simulink model "Test"  (R2026a)
settings: Solver=FixedStepDiscrete  FixedStep=1/200
undefined symbols (not defined in the file or in its folder): position, timestamp, x, y, z
libraries: px4_lib x33, dspsigops x3
settings Model: Creator=jack  LastModifiedBy=jack
settings OptimizationCC: DefaultUnderspecifiedDataType=single
settings DebuggingCC: ParameterPrecisionLossMsg=none
settings HardwareCC: ProdBitPerLong=64.0  ProdHWDeviceType=Intel->x86-64 (Linux 64)
settings SFSimCC: SimCustomHeaderCode="#include \"px4_simulink_api.h\""  SimUserSources=px4_simulink_api.cpp  SimTargetLang=C++
settings RTWCC: SystemTargetFile=ert.tlc  GenCodeOnly=on  PostCodeGenCommand=px4API.runPostCodeGen(buildInfo)  CustomHeaderCode="#include \"px4_simulink_api.h\""  Toolchain=GNU Tools for PX4 Autopilots  DataTypeReplacement=CDataTypesFixedWidth  TargetLang=C++  Description=Embedded Coder
settings ERTTargetCC: ExtModeTransport=2.0  RootIOFormat=Structure reference  MaxIdInt64=INT64_MAX  MinIdInt64=INT64_MIN  MaxIdUint64=UINT64_MAX  MaxIdInt32=INT32_MAX  MinIdInt32=INT32_MIN  MaxIdUint32=UINT32_MAX  MaxIdInt16=INT16_MAX  MinIdInt16=INT16_MIN  MaxIdUint16=UINT16_MAX  MaxIdInt8=INT8_MAX  MinIdInt8=INT8_MIN  MaxIdUint8=UINT8_MAX  TargetLangStandard=C++14 (ISO)  CodeInterfacePackaging=C++ class  SubcomponentCodeInterfacePackaging=C++ class

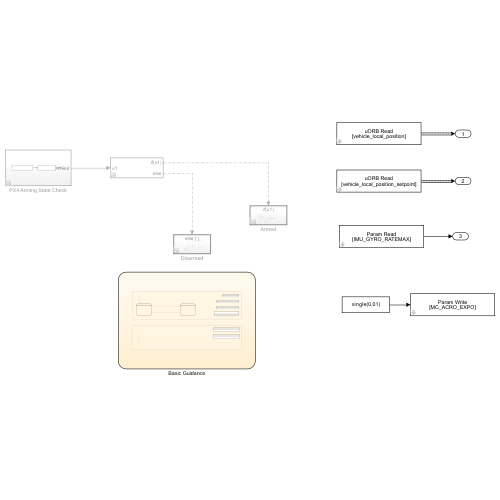
[thumbnail: Simulink's stored preview of the top-level diagram]
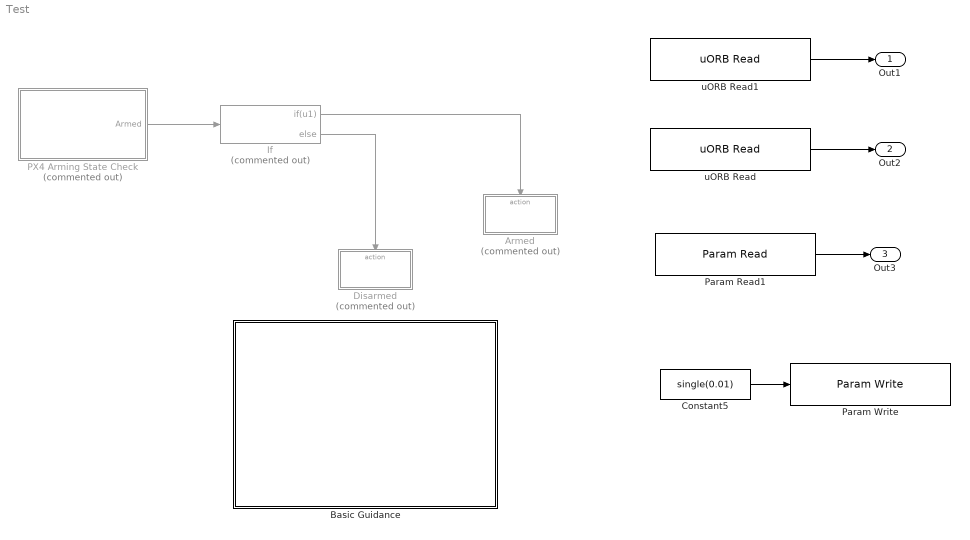
== system Test ==
  Armed : Subsystem  Commented=on  TreatAsAtomicUnit=on
  Basic Guidance : Stateflow chart  TreatAsAtomicUnit=on
  Constant5 : Constant  Value=single(0.01)
  Disarmed : Subsystem  Commented=on  TreatAsAtomicUnit=on
  If : If  Commented=on  IfExpression=u1
  PX4 Arming State Check : Subsystem  Commented=on
  Param Read1 : px4_lib/Param Read  param_name=IMU_GYRO_RATEMAX  param_type=int32  sample_time=-1
  Param Write : px4_lib/Param Write  param_name=MC_ACRO_EXPO  param_type=single  sample_time=1/5
  uORB Read : px4_lib/uORB Read  uorb_topic=vehicle_local_position_setpoint  sample_time=1/200
  uORB Read1 : px4_lib/uORB Read  uorb_topic=vehicle_local_position  sample_time=1/200
  Out1 : Outport
  Out2 : Outport  Port=2
  Out3 : Outport  Port=3
  wires:
  uORB Read1/1 -> Out1/1
  uORB Read/1 -> Out2/1
  Param Read1/1 -> Out3/1
  Constant5/1 -> Param Write/1
  PX4 Arming State Check/1(Armed) -> If/1
  If/1 -> Armed/Action
  If/2 -> Disarmed/Action

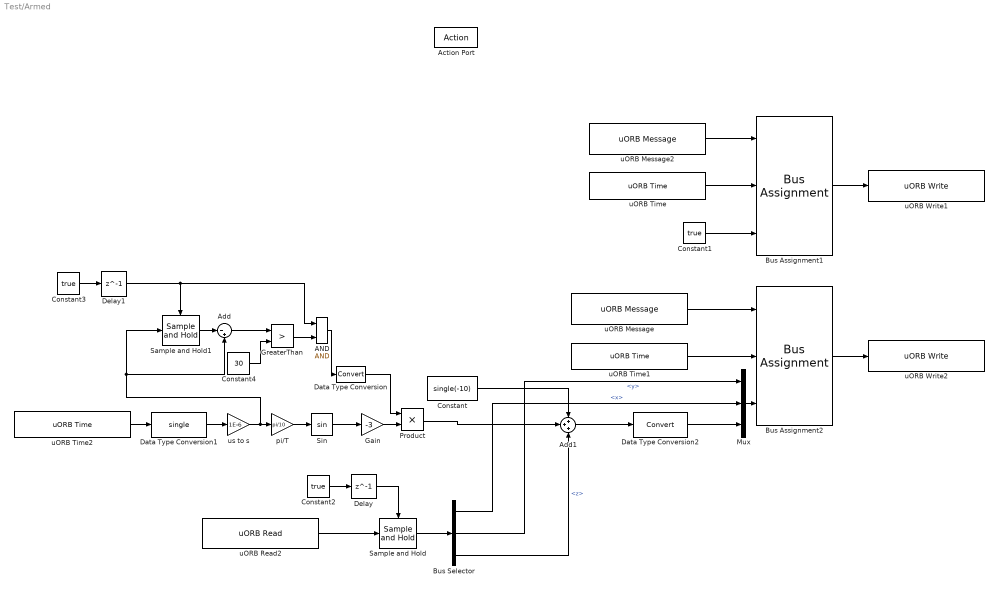
== system Test/Armed ==
  Action Port : ActionPort  InitializeStates=reset  ActionPortLabel=if(u1)
  AND : Logic  IconShape=distinctive  AllPortsSameDT=off  OutDataTypeStr=boolean
  Add : Sum  Inputs=|-+
  Add1 : Sum  Inputs=+++
  Bus Assignment1 : BusAssignment  AssignedSignals=timestamp,position
  Bus Assignment2 : BusAssignment  AssignedSignals=timestamp,position
  Bus Selector : BusSelector  OutputSignals=x,y,z
  Constant : Constant  Value=single(-10)
  Constant1 : Constant  Value=true
  Constant2 : Constant  Value=true
  Constant3 : Constant  Value=true
  Constant4 : Constant  Value=30
  Data Type Conversion : DataTypeConversion  SaturateOnIntegerOverflow=off  RndMeth=Floor
  Data Type Conversion1 : DataTypeConversion  OutDataTypeStr=single  SaturateOnIntegerOverflow=off  RndMeth=Floor
  Data Type Conversion2 : DataTypeConversion  SaturateOnIntegerOverflow=off  RndMeth=Floor
  Delay : Delay  DelayLength=1  InitialCondition=false
  Delay1 : Delay  DelayLength=1  InitialCondition=false
  Gain : Gain  Gain=-3  ParamDataTypeStr=single
  GreaterThan : RelationalOperator  Operator=>  OutDataTypeStr=boolean  RndMeth=Simplest  InputSameDT=off
  Mux : Mux  Inputs=3
  Product : Product
  Sample and Hold : dspsigops/Sample and Hold  trig=Rising edge  initCond=0  latchinput=off
  Sample and Hold1 : dspsigops/Sample and Hold  trig=Rising edge  initCond=0  latchinput=off
  Sin : Trigonometry  OutputSignalType=real
  pi/T : Gain  Gain=pi/10  ParamDataTypeStr=single
  uORB Message : px4_lib/uORB Message  uorb_topic=trajectory_setpoint6dof  sample_time=-1  init_value=NaN
  uORB Message2 : px4_lib/uORB Message  uorb_topic=offboard_control_mode  sample_time=-1  init_value=0
  uORB Read2 : px4_lib/uORB Read  uorb_topic=vehicle_local_position_setpoint  sample_time=-1
  uORB Time : px4_lib/uORB Time  sample_time=-1
  uORB Time1 : px4_lib/uORB Time  sample_time=-1
  uORB Time2 : px4_lib/uORB Time  sample_time=-1
  uORB Write1 : px4_lib/uORB Write  uorb_topic=offboard_control_mode  sample_time=1/50
  uORB Write2 : px4_lib/uORB Write  uorb_topic=vehicle_local_position_setpoint  sample_time=1/50
  us to s : Gain  Gain=1E-6  ParamDataTypeStr=single
  wires:
  uORB Message/1 -> Bus Assignment2/1
  uORB Time/1 -> Bus Assignment1/2
  Bus Selector/3 -> Add1/3  "<z>"
  Bus Selector/2 -> Mux/1  "<y>"
  Mux/1 -> Bus Assignment2/3
  uORB Time1/1 -> Bus Assignment2/2
  pi/T/1 -> Sin/1
  Constant/1 -> Add1/1
  Gain/1 -> Product/2
  Bus Assignment1/1 -> uORB Write1/1
  uORB Message2/1 -> Bus Assignment1/1
  GreaterThan/1 -> AND/2
  Constant2/1 -> Delay/1
  Delay1/1 -> AND/1, Sample and Hold1/Trigger
  Sample and Hold1/1 -> Add/1
  Sin/1 -> Gain/1
  Bus Assignment2/1 -> uORB Write2/1
  Constant1/1 -> Bus Assignment1/3
  Add1/1 -> Data Type Conversion2/1
  Delay/1 -> Sample and Hold/Trigger
  Add/1 -> GreaterThan/1
  Product/1 -> Add1/2
  Data Type Conversion2/1 -> Mux/3
  Data Type Conversion/1 -> Product/1
  AND/1 -> Data Type Conversion/1
  Data Type Conversion1/1 -> us to s/1
  Constant3/1 -> Delay1/1
  uORB Time2/1 -> Data Type Conversion1/1
  us to s/1 -> Add/2, Sample and Hold1/1, pi/T/1
  Bus Selector/1 -> Mux/2  "<x>"
  Sample and Hold/1 -> Bus Selector/1
  uORB Read2/1 -> Sample and Hold/1
  Constant4/1 -> GreaterThan/2

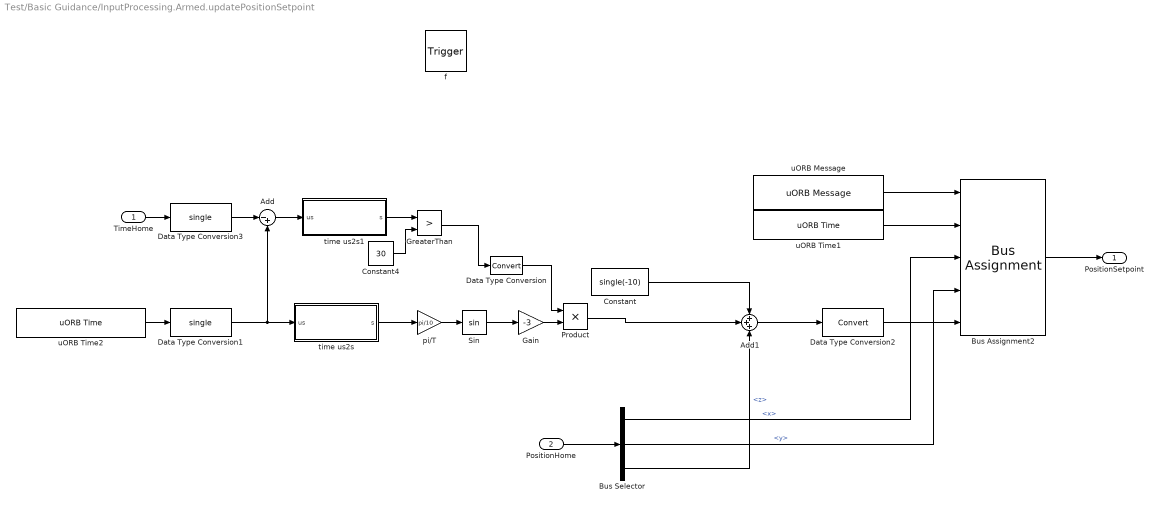
== system Test/Basic Guidance/InputProcessing.Armed.updatePositionSetpoint ==
  TimeHome : Inport  OutDataTypeStr=uint64  PortDimensions=1
  PositionHome : Inport  Port=2  OutDataTypeStr=Bus: vehicle_local_position_s  PortDimensions=1
  f : TriggerPort  TriggerType=function-call  VariantControl=(inherit)
      settings: CopyFcn=Stateflow.SLINSF.SimulinkMan.removeBlockPreDeleteFcn  PreDeleteFcn=Stateflow.SLINSF.SimulinkMan.unsafePredeleteFcn
  Add : Sum  Inputs=|-+
  Add1 : Sum  Inputs=+++
  Bus Assignment2 : BusAssignment  AssignedSignals=timestamp,x,y,z
  Bus Selector : BusSelector  OutputSignals=x,y,z
  Constant : Constant  Value=single(-10)
  Constant4 : Constant  Value=30
  Data Type Conversion : DataTypeConversion  SaturateOnIntegerOverflow=off  RndMeth=Floor
  Data Type Conversion1 : DataTypeConversion  OutDataTypeStr=single  SaturateOnIntegerOverflow=off  RndMeth=Floor
  Data Type Conversion2 : DataTypeConversion  SaturateOnIntegerOverflow=off  RndMeth=Floor
  Data Type Conversion3 : DataTypeConversion  OutDataTypeStr=single  SaturateOnIntegerOverflow=off  RndMeth=Floor
  Gain : Gain  Gain=-3  ParamDataTypeStr=single
  GreaterThan : RelationalOperator  Operator=>  OutDataTypeStr=boolean  RndMeth=Simplest  InputSameDT=off
  Product : Product
  Sin : Trigonometry  OutputSignalType=real
  pi/T : Gain  Gain=pi/10  ParamDataTypeStr=single
  time us2s : Subsystem
  time us2s1 : Subsystem
  uORB Message : px4_lib/uORB Message  uorb_topic=vehicle_local_position_setpoint  sample_time=-1  init_value=NaN
  uORB Time1 : px4_lib/uORB Time  sample_time=-1
  uORB Time2 : px4_lib/uORB Time  sample_time=-1
  PositionSetpoint : Outport  OutDataTypeStr=Bus: vehicle_local_position_setpoint_s  PortDimensions=1
  wires:
  Constant/1 -> Add1/1
  uORB Time2/1 -> Data Type Conversion1/1
  Add1/1 -> Data Type Conversion2/1
  uORB Message/1 -> Bus Assignment2/1
  TimeHome/1 -> Data Type Conversion3/1
  pi/T/1 -> Sin/1
  Data Type Conversion/1 -> Product/1
  Data Type Conversion2/1 -> Bus Assignment2/5
  uORB Time1/1 -> Bus Assignment2/2
  Constant4/1 -> GreaterThan/2
  Add/1 -> time us2s1/1(us)
  Product/1 -> Add1/2
  time us2s/1(s) -> pi/T/1
  GreaterThan/1 -> Data Type Conversion/1
  Gain/1 -> Product/2
  Sin/1 -> Gain/1
  Bus Selector/3 -> Add1/3  "<z>"
  Bus Assignment2/1 -> PositionSetpoint/1
  time us2s1/1(s) -> GreaterThan/1
  PositionHome/1 -> Bus Selector/1
  Bus Selector/2 -> Bus Assignment2/4  "<y>"
  Bus Selector/1 -> Bus Assignment2/3  "<x>"
  Data Type Conversion1/1 -> time us2s/1(us), Add/2
  Data Type Conversion3/1 -> Add/1

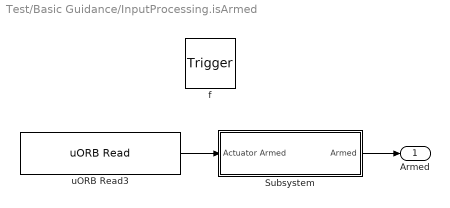
== system Test/Basic Guidance/InputProcessing.isArmed ==
  f : TriggerPort  TriggerType=function-call  VariantControl=(inherit)
      settings: CopyFcn=Stateflow.SLINSF.SimulinkMan.removeBlockPreDeleteFcn  PreDeleteFcn=Stateflow.SLINSF.SimulinkMan.unsafePredeleteFcn
  Subsystem : Subsystem
  uORB Read3 : px4_lib/uORB Read  uorb_topic=actuator_armed  sample_time=-1
  Armed : Outport
  wires:
  uORB Read3/1 -> Subsystem/1(Actuator Armed)
  Subsystem/1(Armed) -> Armed/1

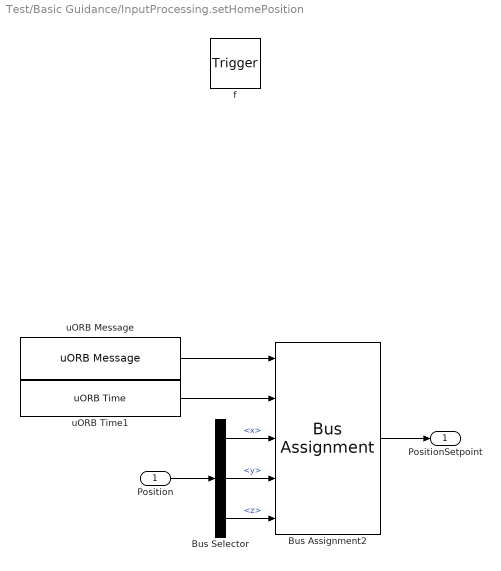
== system Test/Basic Guidance/InputProcessing.setHomePosition ==
  Position : Inport  OutDataTypeStr=Bus: vehicle_local_position_s  PortDimensions=1
  f : TriggerPort  TriggerType=function-call  VariantControl=(inherit)
      settings: CopyFcn=Stateflow.SLINSF.SimulinkMan.removeBlockPreDeleteFcn  PreDeleteFcn=Stateflow.SLINSF.SimulinkMan.unsafePredeleteFcn
  Bus Assignment2 : BusAssignment  AssignedSignals=timestamp,x,y,z
  Bus Selector : BusSelector  OutputSignals=x,y,z
  uORB Message : px4_lib/uORB Message  uorb_topic=vehicle_local_position_setpoint  sample_time=-1  init_value=NaN
  uORB Time1 : px4_lib/uORB Time  sample_time=-1
  PositionSetpoint : Outport
  wires:
  uORB Message/1 -> Bus Assignment2/1
  Bus Assignment2/1 -> PositionSetpoint/1
  uORB Time1/1 -> Bus Assignment2/2
  Position/1 -> Bus Selector/1
  Bus Selector/3 -> Bus Assignment2/5  "<z>"
  Bus Selector/2 -> Bus Assignment2/4  "<y>"
  Bus Selector/1 -> Bus Assignment2/3  "<x>"

== system Test/Basic Guidance/InputProcessing.time ==
  f : TriggerPort  TriggerType=function-call  VariantControl=(inherit)
      settings: CopyFcn=Stateflow.SLINSF.SimulinkMan.removeBlockPreDeleteFcn  PreDeleteFcn=Stateflow.SLINSF.SimulinkMan.unsafePredeleteFcn
  uORB Time2 : px4_lib/uORB Time  sample_time=-1
  t : Outport  OutDataTypeStr=uint64
  wires:
  uORB Time2/1 -> t/1

== system Test/Basic Guidance/InputProcessing.updatePosition ==
  f : TriggerPort  TriggerType=function-call  VariantControl=(inherit)
      settings: CopyFcn=Stateflow.SLINSF.SimulinkMan.removeBlockPreDeleteFcn  PreDeleteFcn=Stateflow.SLINSF.SimulinkMan.unsafePredeleteFcn
  uORB Read2 : px4_lib/uORB Read  uorb_topic=vehicle_local_position  sample_time=-1
  Position : Outport
  wires:
  uORB Read2/1 -> Position/1

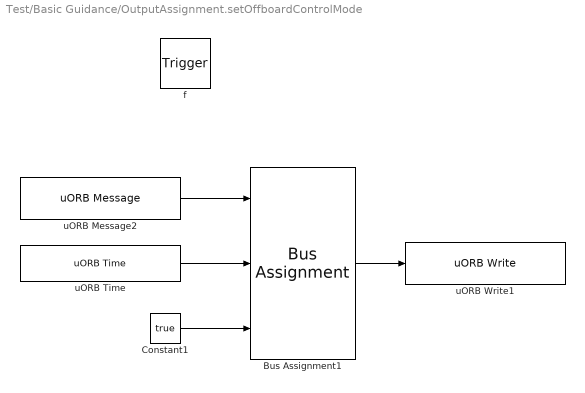
== system Test/Basic Guidance/OutputAssignment.setOffboardControlMode ==
  f : TriggerPort  TriggerType=function-call  VariantControl=(inherit)
      settings: CopyFcn=Stateflow.SLINSF.SimulinkMan.removeBlockPreDeleteFcn  PreDeleteFcn=Stateflow.SLINSF.SimulinkMan.unsafePredeleteFcn
  Bus Assignment1 : BusAssignment  AssignedSignals=timestamp,position
  Constant1 : Constant  Value=true
  uORB Message2 : px4_lib/uORB Message  uorb_topic=offboard_control_mode  sample_time=-1  init_value=0
  uORB Time : px4_lib/uORB Time  sample_time=-1
  uORB Write1 : px4_lib/uORB Write  uorb_topic=offboard_control_mode  sample_time=-1
  wires:
  uORB Time/1 -> Bus Assignment1/2
  Constant1/1 -> Bus Assignment1/3
  Bus Assignment1/1 -> uORB Write1/1
  uORB Message2/1 -> Bus Assignment1/1

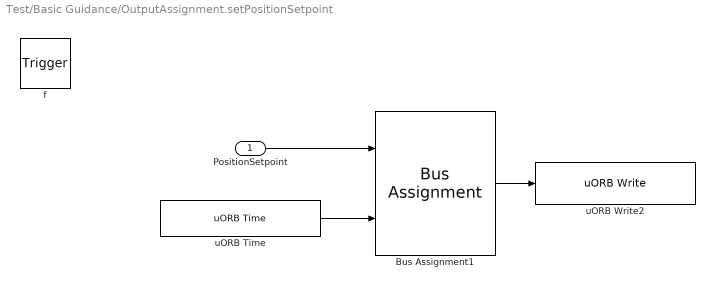
== system Test/Basic Guidance/OutputAssignment.setPositionSetpoint ==
  PositionSetpoint : Inport  OutDataTypeStr=Bus: vehicle_local_position_setpoint_s  PortDimensions=1
  f : TriggerPort  TriggerType=function-call  VariantControl=(inherit)
      settings: CopyFcn=Stateflow.SLINSF.SimulinkMan.removeBlockPreDeleteFcn  PreDeleteFcn=Stateflow.SLINSF.SimulinkMan.unsafePredeleteFcn
  Bus Assignment1 : BusAssignment  AssignedSignals=timestamp
  uORB Time : px4_lib/uORB Time  sample_time=-1
  uORB Write2 : px4_lib/uORB Write  uorb_topic=vehicle_local_position_setpoint  sample_time=-1
  wires:
  uORB Time/1 -> Bus Assignment1/2
  PositionSetpoint/1 -> Bus Assignment1/1
  Bus Assignment1/1 -> uORB Write2/1

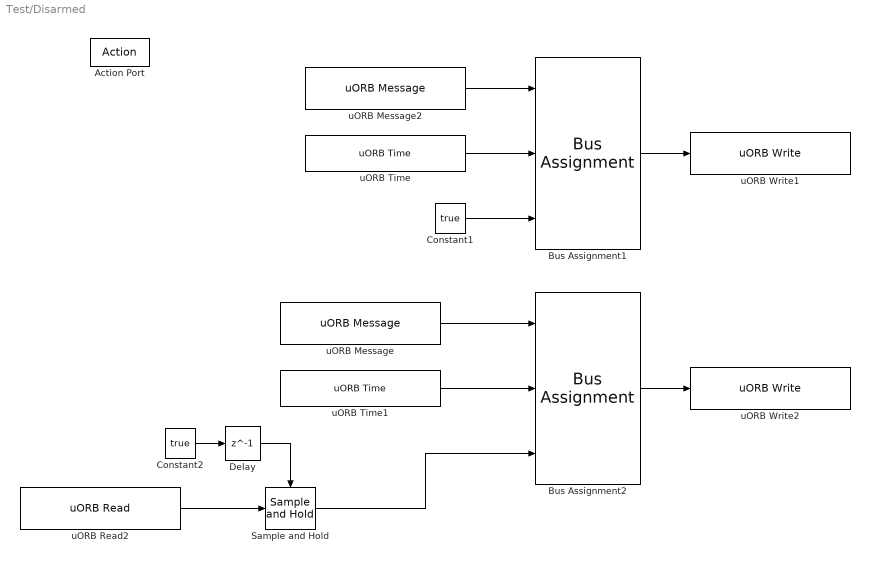
== system Test/Disarmed ==
  Action Port : ActionPort  ActionPortLabel=else
  Bus Assignment1 : BusAssignment  AssignedSignals=timestamp,position
  Bus Assignment2 : BusAssignment  AssignedSignals=timestamp,position
  Constant1 : Constant  Value=true
  Constant2 : Constant  Value=true
  Delay : Delay  DelayLength=1  InitialCondition=false
  Sample and Hold : dspsigops/Sample and Hold  trig=Rising edge  initCond=0  latchinput=off
  uORB Message : px4_lib/uORB Message  uorb_topic=trajectory_setpoint6dof  sample_time=-1  init_value=NaN
  uORB Message2 : px4_lib/uORB Message  uorb_topic=offboard_control_mode  sample_time=-1  init_value=0
  uORB Read2 : px4_lib/uORB Read  uorb_topic=vehicle_local_position_setpoint  sample_time=-1
  uORB Time : px4_lib/uORB Time  sample_time=-1
  uORB Time1 : px4_lib/uORB Time  sample_time=-1
  uORB Write1 : px4_lib/uORB Write  uorb_topic=offboard_control_mode  sample_time=1/50
  uORB Write2 : px4_lib/uORB Write  uorb_topic=trajectory_setpoint6dof  sample_time=1/50
  wires:
  uORB Message/1 -> Bus Assignment2/1
  uORB Time/1 -> Bus Assignment1/2
  uORB Time1/1 -> Bus Assignment2/2
  Bus Assignment1/1 -> uORB Write1/1
  uORB Message2/1 -> Bus Assignment1/1
  Constant2/1 -> Delay/1
  Bus Assignment2/1 -> uORB Write2/1
  Constant1/1 -> Bus Assignment1/3
  Delay/1 -> Sample and Hold/Trigger
  uORB Read2/1 -> Sample and Hold/1
  Sample and Hold/1 -> Bus Assignment2/3

== system Test/PX4 Arming State Check ==
  Subsystem : Subsystem
  uORB Read3 : px4_lib/uORB Read  uorb_topic=actuator_armed  sample_time=1/800
  Armed : Outport
  wires:
  uORB Read3/1 -> Subsystem/1(Actuator Armed)
  Subsystem/1(Armed) -> Armed/1

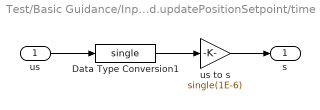
== system Test/Basic Guidance/InputProcessing.Armed.updatePositionSetpoint/time us2s ==
  us : Inport
  Data Type Conversion1 : DataTypeConversion  OutDataTypeStr=single  SaturateOnIntegerOverflow=off  RndMeth=Floor
  us to s : Gain  Gain=single(1E-6)  ParamDataTypeStr=single
  s : Outport
  wires:
  Data Type Conversion1/1 -> us to s/1
  us/1 -> Data Type Conversion1/1
  us to s/1 -> s/1

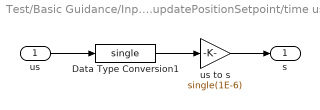
== system Test/Basic Guidance/InputProcessing.Armed.updatePositionSetpoint/time us2s1 ==
  us : Inport
  Data Type Conversion1 : DataTypeConversion  OutDataTypeStr=single  SaturateOnIntegerOverflow=off  RndMeth=Floor
  us to s : Gain  Gain=single(1E-6)  ParamDataTypeStr=single
  s : Outport
  wires:
  us to s/1 -> s/1
  us/1 -> Data Type Conversion1/1
  Data Type Conversion1/1 -> us to s/1

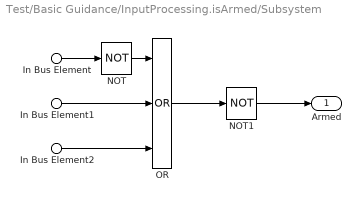
== system Test/Basic Guidance/InputProcessing.isArmed/Subsystem ==
  In Bus Element : Inport  PortName=Actuator Armed  Element=armed
  In Bus Element1 : Inport  PortName=Actuator Armed  Element=lockdown
  In Bus Element2 : Inport  PortName=Actuator Armed  Element=in_esc_calibration_mode
  NOT : Logic  Operator=NOT  IconShape=distinctive  AllPortsSameDT=off  OutDataTypeStr=boolean
  NOT1 : Logic  Operator=NOT  IconShape=distinctive  AllPortsSameDT=off  OutDataTypeStr=boolean
  OR : Logic  Operator=OR  Inputs=3  IconShape=distinctive  AllPortsSameDT=off  OutDataTypeStr=boolean
  Armed : Outport
  wires:
  NOT1/1 -> Armed/1
  In Bus Element/1 -> NOT/1
  In Bus Element1/1 -> OR/2
  In Bus Element2/1 -> OR/3
  NOT/1 -> OR/1
  OR/1 -> NOT1/1

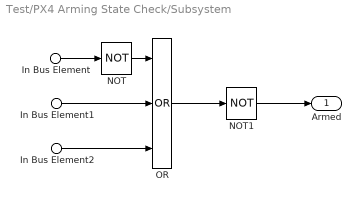
== system Test/PX4 Arming State Check/Subsystem ==
  In Bus Element : Inport  PortName=Actuator Armed  Element=armed
  In Bus Element1 : Inport  PortName=Actuator Armed  Element=lockdown
  In Bus Element2 : Inport  PortName=Actuator Armed  Element=in_esc_calibration_mode
  NOT : Logic  Operator=NOT  IconShape=distinctive  AllPortsSameDT=off  OutDataTypeStr=boolean
  NOT1 : Logic  Operator=NOT  IconShape=distinctive  AllPortsSameDT=off  OutDataTypeStr=boolean
  OR : Logic  Operator=OR  Inputs=3  IconShape=distinctive  AllPortsSameDT=off  OutDataTypeStr=boolean
  Armed : Outport
  wires:
  NOT1/1 -> Armed/1
  In Bus Element/1 -> NOT/1
  In Bus Element1/1 -> OR/2
  In Bus Element2/1 -> OR/3
  NOT/1 -> OR/1
  OR/1 -> NOT1/1

== stateflow chart Test/Basic Guidance ==
  settings: updateMethod=DISCRETE  sampleTime=1/200
  state InputProcessing [parallel]
    settings: executionOrder=1
    state t = time [function]
    state Armed = isArmed [function]
    state Armed
      state PositionSetpoint = updatePositionSetpoint(TimeHome,PositionHome) [function]
      (default) -> (junction 51) : {
          | PositionSetpoint = updatePositionSetpoint(TimeHome, PositionHome);
          | }
    state Disarmed
    state Position = updatePosition [function]
    state PositionSetpoint = setHomePosition(Position) [function]
    (default) -> Disarmed : {
        | TimeHome = time();
        | PositionHome = updatePosition();
        | PositionSetpoint = setHomePosition(PositionHome);
        | }
    Disarmed -> Armed : [isArmed()]{
        | TimeHome = time();
        | PositionHome = updatePosition();
        | }
    Armed -> Disarmed : [~isArmed()]
  state OutputAssignment [parallel]
    settings: executionOrder=2
    state setOffboardControlMode [function]
    state setPositionSetpoint(PositionSetpoint) [function]
    (default) -> (junction 37) : {
        | setOffboardControlMode();
        | setPositionSetpoint(PositionSetpoint);
        | }
  data: t function_output uint64; Armed function_output; TimeHome function_input uint64 size=1; PositionHome function_input Bus: vehicle_local_position_s size=1; PositionSetpoint function_output Bus: vehicle_local_position_setpoint_s size=1; Position function_output; PositionSetpoint function_output; Position function_input Bus: vehicle_local_position_s size=1; PositionSetpoint function_input Bus: vehicle_local_position_setpoint_s size=1; PositionHome local Bus: vehicle_local_position_s size=1; PositionSetpoint local Bus: vehicle_local_position_setpoint_s size=1; TimeHome local size=1
